simulink model "LaserSim"  (R2020a)
settings: Solver=VariableStepAuto  StartTime=0.0  StopTime=Tsim  RelTol=1e-3
values from neighbouring files (symbols this model uses):
  A1 = 1    [Laser.m]
  A2 = 0    [Laser.m]
  A3 = 0    [Laser.m]
  A4 = 0    [Laser.m]
  A5 = 0    [Laser.m]
  A6 = 0    [Laser.m]
  F1 = 85000    [Laser.m]
  F2 = 90000    [Laser.m]
  F3 = 95000    [Laser.m]
  F4 = 100000    [Laser.m]
  F5 = 115000    [Laser.m]
  F6 = 120000    [Laser.m]
  Te = T/M    (= 3.125e-06)    [Laser.m]    (also in scriptDFT.m)
  Tsim = T-Te    (= 0.000196875)    [Laser.m]    (also in scriptDFT.m)
settings Model: Creator=mvacher  LastModifiedBy=mvacher

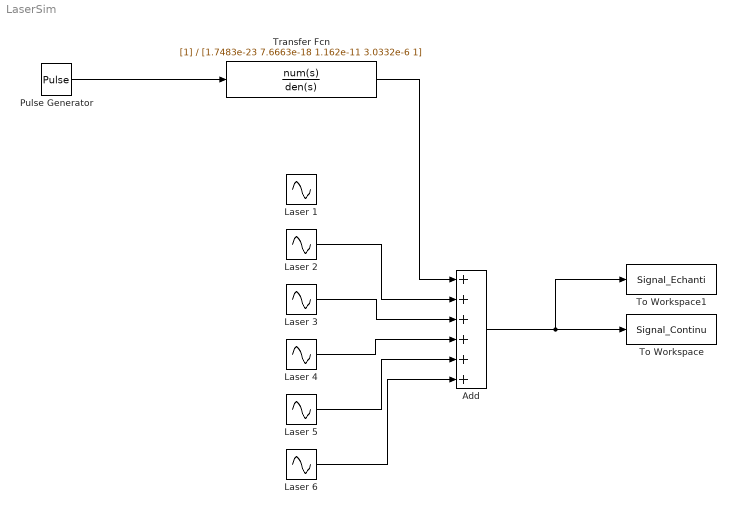
== system LaserSim ==
  Add : Sum  Inputs=++++++
  Laser 1 : Sin  Amplitude=A1  Frequency=2*pi*F1  SampleTime=0
  Laser 2 : Sin  Amplitude=A2  Frequency=2*pi*F2  SampleTime=0
  Laser 3 : Sin  Amplitude=A3  Frequency=2*pi*F3  SampleTime=0
  Laser 4 : Sin  Amplitude=A4  Frequency=2*pi*F4  SampleTime=0
  Laser 5 : Sin  Amplitude=A5  Frequency=2*pi*F5  SampleTime=0
  Laser 6 : Sin  Amplitude=A6  Frequency=2*pi*F6  SampleTime=0
  Pulse Generator : DiscretePulseGenerator  PulseType=Time based  Amplitude=A1  Period=1/F1  PulseWidth=50
  To Workspace : ToWorkspace  VariableName=Signal_Continu  SaveFormat=Timeseries  SampleTime=Tsim/1000
  To Workspace1 : ToWorkspace  VariableName=Signal_Echanti  SaveFormat=Timeseries  SampleTime=Te
  Transfer Fcn : TransferFcn  Denominator=[1.7483e-23 7.6663e-18 1.162e-11 3.0332e-6 1]
  wires:
  Laser 2/1 -> Add/2
  Laser 3/1 -> Add/3
  Laser 4/1 -> Add/4
  Laser 5/1 -> Add/5
  Laser 6/1 -> Add/6
  Add/1 -> To Workspace/1, To Workspace1/1
  Pulse Generator/1 -> Transfer Fcn/1
  Transfer Fcn/1 -> Add/1
